simulink model "SmoothSetPoint"  (R2016b)
settings: Solver=FixedStepAuto  StartTime=0.0  StopTime=10.0  RelTol=1e-3  EnableMultiTasking=on
libraries: simulink x1
settings Model: Creator=march  LastModifiedBy=march
settings SolverCC: EnableConcurrentExecution=on
settings DataIOCC: SaveFormat=StructureWithTime
settings OptimizationCC: BlockReduction=off  OptimizeBlockIOStorage=off  BufferReuse=off  GlobalBufferReuse=off  ExpressionFolding=off  LocalBlockOutputs=off
settings HardwareCC: ProdBitPerPointer=32  ProdBitPerSizeT=32  ProdBitPerPtrDiffT=32  ProdLargestAtomicFloat=None  ProdWordSize=32  ProdLongLongMode=on  ProdHWDeviceType=Generic->32-bit x86 compatible
settings RTWCC: SystemTargetFile=slrt.tlc  TemplateMakefile=slrt_default_tmf  Description=Simulink Real-Time  RTWCompilerOptimization=on

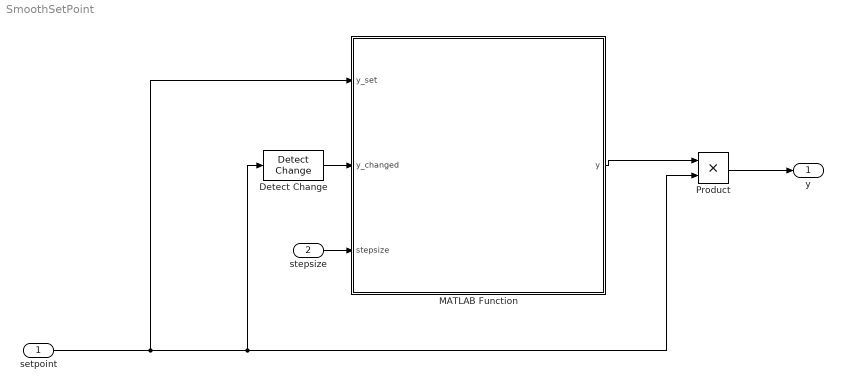
== system SmoothSetPoint ==
  setpoint : Inport
  stepsize : Inport  Port=2
  Detect Change : simulink/Logic and Bit Operations/Detect Change  vinit=0  OutDataTypeStr=boolean
  MATLAB Function : MATLAB Function  TreatAsAtomicUnit=on
  Product : Product
  y : Outport
  wires:
  MATLAB Function/1(y) -> Product/1
  Product/1 -> y/1
  setpoint/1 -> MATLAB Function/1(y_set), Detect Change/1, Product/2
  Detect Change/1 -> MATLAB Function/2(y_changed)
  stepsize/1 -> MATLAB Function/3(stepsize)

== matlab function SmoothSetPoint/MATLAB Function ==
  data: y_set input; y_changed input; y output; stepsize input
function y = smoothsetpoint(y_set,y_changed,stepsize)
    persistent step
    if isempty(step) || y_changed 
        step = 0;
    end
    
    step = step + stepsize;
    
    y = smoothstep(step,0,y_set);

function y = smoothstep(x,edge0,edge1)
% Approximates x with a smooth step function to avoid too high set points
% https://en.wikipedia.org/wiki/Smoothstep
a = clamp((x-edge0)/(edge1-edge0),0,1);
y = a^2*(3-2*a);

function y = clamp(x,lower_limit,upper_limit)
    y = x;
    if x < lower_limit 
        y = lower_limit;
    end
    if x > upper_limit
        y = upper_limit;
    end
